simulink model "sol7_PIDFeed"  (R2021b)
settings: Solver=VariableStepAuto  StartTime=0.0  StopTime=5  RelTol=1e-3
PreLoadFcn:
  | initModelData
  | trajectoryData
  | controlPID
StartFcn:
  | controlPID
values from neighbouring files (symbols this model uses):
  B = Bm+(Kb*Km/R)    (= 0.0149065789474)    [MyData_for_1_and_2.m]    (also in MyData_for_3_4_and_5.m; MyData_for_5_and_6.m)
  Jm = 5.5e-4    (= 0.00055)    [MyData_for_1_and_2.m]    (also in MyData_for_3_4_and_5.m; MyData_for_5_and_6.m)
  Kd = (R/Km)*((2*Jm*w*zeta)-B)    (= 0.369819047619)    [MyData_for_1_and_2.m]    (also in MyData_for_3_4_and_5.m = 0.2902; MyData_for_5_and_6.m = 0.0513428571429)
  Km = 0.105    [MyData_for_1_and_2.m]    (also in MyData_for_3_4_and_5.m; MyData_for_5_and_6.m)
  Kp = (R/Km)*(Jm*(w^2))    (= 14.3314285714)    [MyData_for_1_and_2.m]    (also in MyData_for_3_4_and_5.m = 9.95238095238; MyData_for_5_and_6.m = 1.59238095238)
  R = 0.76    [MyData_for_1_and_2.m]    (also in MyData_for_3_4_and_5.m; MyData_for_5_and_6.m)
  r = 156    [MyData_for_1_and_2.m]    (also in MyData_for_3_4_and_5.m; MyData_for_5_and_6.m)
undefined symbols (not defined in the file or in its folder): Ki
settings Model: Creator=esdan  LastModifiedBy=munir
settings SolverCC: AlgebraicLoopSolver=TrustRegion
settings DebuggingCC: SFMachineParentedDataDiag=warning

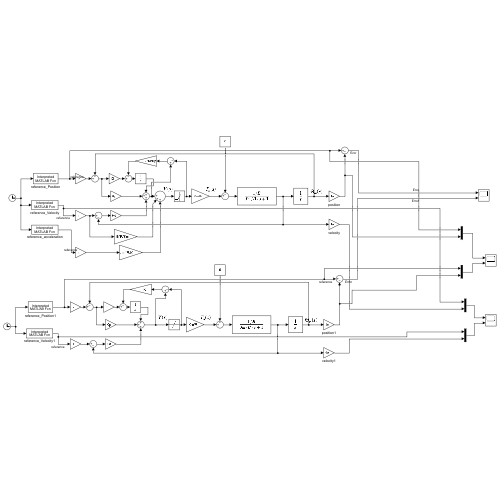
[thumbnail: Simulink's stored preview of the top-level diagram]
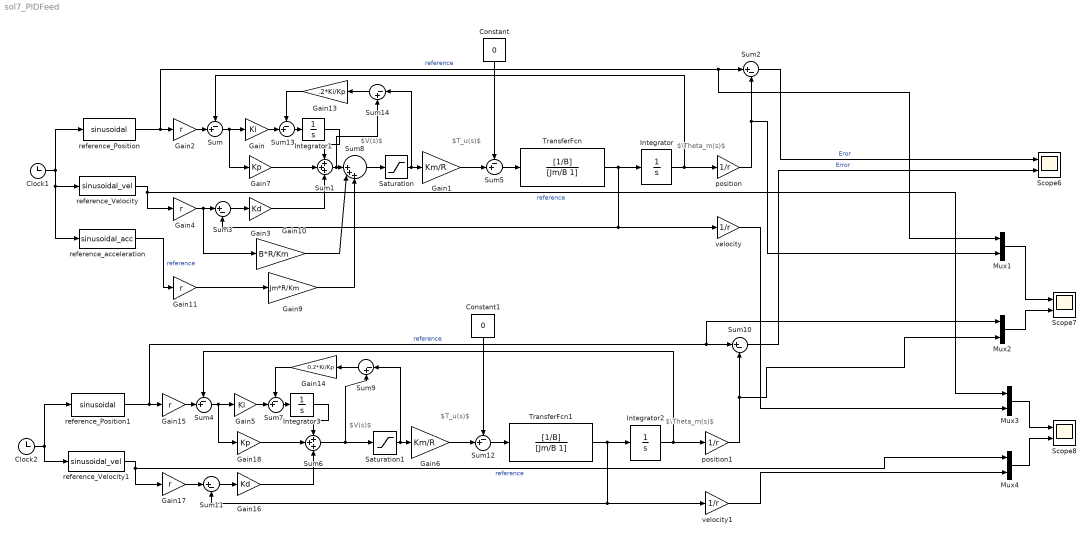
== system sol7_PIDFeed ==
  note: $\Theta_m(s)$
  note: $V(s)$
  note: $T_u(s)$
  note: $V(s)$
  note: $\Theta_m(s)$
  note: $T_u(s)$
  Clock1 : Clock
  Clock2 : Clock
  Constant : Constant  Value=0
  Constant1 : Constant  Value=0
  Gain : Gain  Gain=Ki
  Gain1 : Gain  Gain=Km/R
  Gain10 : Gain  Gain=B*R/Km
  Gain{2,4,11,15,17} (5 alike) : Gain  Gain=r
  Gain13 : Gain  Gain=.2*Ki/Kp
  Gain14 : Gain  Gain=0.2*Ki/Kp
  Gain16 : Gain  Gain=Kd
  Gain18 : Gain  Gain=Kp
  Gain3 : Gain  Gain=Kd
  Gain5 : Gain  Gain=Ki
  Gain6 : Gain  Gain=Km/R
  Gain7 : Gain  Gain=Kp
  Gain9 : Gain  Gain=Jm*R/Km
  Integrator{,1..3} (4 alike) : Integrator
  Mux{1..4} (4 alike) : Mux  Inputs=2
  Saturation : Saturate  UpperLimit=35  LowerLimit=-35
  Saturation1 : Saturate  UpperLimit=35  LowerLimit=-35
  Scope6 : Scope  NumInputPorts=2
  Scope7 : Scope  NumInputPorts=2
  Scope8 : Scope  NumInputPorts=2
  Sum{,4..5,7,12..13} (6 alike) : Sum  Inputs=-+|
  Sum1 : Sum  Inputs=+++
  Sum{2..3,10..11} (4 alike) : Sum  Inputs=|+-
  Sum14 : Sum  Inputs=|-+
  Sum6 : Sum  Inputs=+++
  Sum8 : Sum  Inputs=||+++
  Sum9 : Sum  Inputs=|-+
  TransferFcn : TransferFcn  Numerator=[1/B]  Denominator=[Jm/B 1]
  TransferFcn1 : TransferFcn  Numerator=[1/B]  Denominator=[Jm/B 1]
  position : Gain  Gain=1/r
  position1 : Gain  Gain=1/r
  reference_Position : MATLABFcn  MATLABFcn=sinusoidal
  reference_Position1 : MATLABFcn  MATLABFcn=sinusoidal
  reference_Velocity : MATLABFcn  MATLABFcn=sinusoidal_vel
  reference_Velocity1 : MATLABFcn  MATLABFcn=sinusoidal_vel
  reference_acceleration : MATLABFcn  MATLABFcn=sinusoidal_acc
  velocity : Gain  Gain=1/r
  velocity1 : Gain  Gain=1/r
  wires:
  TransferFcn/1 -> Integrator/1, velocity/1, Sum3/2
  Sum/1 -> Gain/1, Gain7/1
  Gain2/1 -> Sum/2
  reference_Position/1 -> Gain2/1, Mux1/1, Sum2/1  "reference"
  Sum3/1 -> Gain3/1
  position/1 -> Mux1/2, Sum2/2
  Integrator/1 -> position/1, Sum/1
  reference_Velocity/1 -> Mux3/1, Gain4/1  "reference"
  Gain4/1 -> Gain10/1, Sum3/1
  Sum5/1 -> TransferFcn/1
  Gain1/1 -> Sum5/2
  Constant/1 -> Sum5/1
  Gain3/1 -> Sum1/3
  Gain7/1 -> Sum1/2
  Integrator1/1 -> Sum1/1
  reference_acceleration/1 -> Gain11/1  "reference"
  Gain11/1 -> Gain9/1
  Gain9/1 -> Sum8/3
  Gain10/1 -> Sum8/2
  Clock1/1 -> reference_Position/1, reference_acceleration/1, reference_Velocity/1
  Sum8/1 -> Saturation/1
  Gain13/1 -> Sum13/1
  Saturation/1 -> Sum14/1, Gain1/1
  Sum14/1 -> Gain13/1
  Sum1/1 -> Sum14/2, Sum8/1
  Gain/1 -> Sum13/2
  Sum13/1 -> Integrator1/1
  Sum2/1 -> Scope6/1  "Eror"
  velocity/1 -> Mux3/2
  Sum10/1 -> Scope6/2  "Error"
  Sum7/1 -> Integrator3/1
  Gain5/1 -> Sum7/2
  reference_Position1/1 -> Gain15/1, Mux2/1, Sum10/1  "reference"
  Saturation1/1 -> Sum9/1, Gain6/1
  velocity1/1 -> Mux4/2
  Integrator2/1 -> position1/1, Sum4/1
  position1/1 -> Mux2/2, Sum10/2
  Gain18/1 -> Sum6/2
  Gain6/1 -> Sum12/2
  Sum11/1 -> Gain16/1
  TransferFcn1/1 -> Integrator2/1, velocity1/1, Sum11/2
  Gain15/1 -> Sum4/2
  Clock2/1 -> reference_Position1/1, reference_Velocity1/1
  Gain17/1 -> Sum11/1
  Integrator3/1 -> Sum6/1
  Sum4/1 -> Gain5/1, Gain18/1
  Constant1/1 -> Sum12/1
  Gain16/1 -> Sum6/3
  Sum12/1 -> TransferFcn1/1
  reference_Velocity1/1 -> Mux4/1, Gain17/1  "reference"
  Sum6/1 -> Sum9/2, Saturation1/1
  Sum9/1 -> Gain14/1
  Gain14/1 -> Sum7/1
  Mux1/1 -> Scope7/1
  Mux2/1 -> Scope7/2
  Mux3/1 -> Scope8/1
  Mux4/1 -> Scope8/2
